simulink subsystem "GlobalPosition"  (R2024b)
settings: Solver=VariableStepAuto  StartTime=0.0  StopTime=10.0  RelTol=1e-3
undefined symbols (not defined in the file or in its folder): Earth, Parameters, WGS84
libraries: aerolibtransform2 x1
settings Model: Creator=thesa  LastModifiedBy=jack

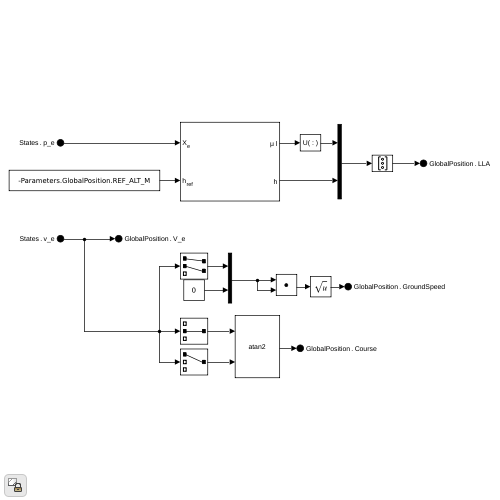
[thumbnail: Simulink's stored preview of the top-level diagram]
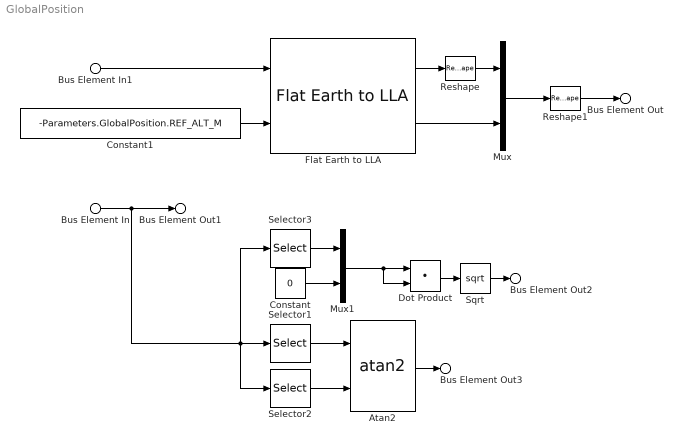
== system GlobalPosition ==
  Bus Element In1 : Inport  PortName=States  Element=p_e
  Bus Element In : Inport  PortName=States  Element=v_e
  Atan2 : Trigonometry  Operator=atan2
  Constant : Constant  Value=0
  Constant1 : Constant  Value=-Parameters.GlobalPosition.REF_ALT_M
  Dot Product : DotProduct  OutDataTypeStr=Inherit: Inherit via internal rule
  Flat Earth to LLA : aerolibtransform2/Flat Earth to LLA  units=Metric (MKS)  ptype=Earth (WGS84)  F=1/298.257223563  R=6378137  refPosPort=off  LL0=[Parameters.GlobalPosition.REF_LAT_DEG, Parameters.GlobalPosition.REF_LONG_DEG]  psi=0
  Mux : Mux  Inputs=2
  Mux1 : Mux  Inputs=2
  Reshape : Reshape
  Reshape1 : Reshape  OutputDimensionality=Column vector (2-D)
  Selector1 : Selector  InputPortWidth=3  IndexOptions=Index vector (dialog)  Indices=2  OutputSizes=1
  Selector2 : Selector  InputPortWidth=3  IndexOptions=Index vector (dialog)  Indices=1  OutputSizes=1
  Selector3 : Selector  InputPortWidth=3  IndexOptions=Index vector (dialog)  Indices=[1,2]  OutputSizes=1
  Sqrt : Sqrt
  Bus Element Out : Outport  PortName=GlobalPosition  Element=LLA
  Bus Element Out1 : Outport  PortName=GlobalPosition  Element=V_e
  Bus Element Out2 : Outport  PortName=GlobalPosition  Element=GroundSpeed
  Bus Element Out3 : Outport  PortName=GlobalPosition  Element=Course
  wires:
  Reshape/1 -> Mux/1
  Flat Earth to LLA/1 -> Reshape/1
  Mux/1 -> Reshape1/1
  Reshape1/1 -> Bus Element Out/1
  Selector2/1 -> Atan2/2
  Selector1/1 -> Atan2/1
  Selector3/1 -> Mux1/1
  Mux1/1 -> Dot Product/1, Dot Product/2
  Dot Product/1 -> Sqrt/1
  Constant/1 -> Mux1/2
  Bus Element In/1 -> Bus Element Out1/1, Selector1/1, Selector3/1, Selector2/1
  Bus Element In1/1 -> Flat Earth to LLA/1
  Sqrt/1 -> Bus Element Out2/1
  Atan2/1 -> Bus Element Out3/1
  Flat Earth to LLA/2 -> Mux/2
  Constant1/1 -> Flat Earth to LLA/2
